simulink model "A5_model_10"  (R2024a)
settings: Solver=VariableStepAuto  StartTime=0.0  StopTime=10  FixedStep=0.00001  MaxStep=1e-3  RelTol=1e-3
values from neighbouring files (symbols this model uses):
  a = data(5)    [A5_41.m]
  A_d = eye(size(A)) + H*(A-(L.*C_Y))    [A5_41.m]
  b = data(6)    [A5_41.m]
  B_d = B * H    [A5_41.m]
  c1 = data(3)    [A5_41.m]
  c2 = data(4)    [A5_41.m]
  h = 0.01    [A5_41.m]
  J_10 = 5220    [A5_41.m]
  K = [S1-temp(2) S2-temp(3) S3-temp(4) S4-temp(5) S5-temp(6)]*Wrtilde*inv(Wr)    [A5_41.m]
  k1 = data(8)    [A5_41.m]
  kr = (-1)/(C_Y*inv(A-B*K)*B)    [A5_41.m]
  L_d = L * H    [A5_41.m]
  m_10 = m+400    [A5_41.m]
  tau = data(7)    [A5_41.m]
  V_10 = 30    [A5_41.m]
settings Model: Creator=jofr  LastModifiedBy=munav
settings SolverCC: AlgebraicLoopSolver=TrustRegion
settings DataIOCC: LimitDataPoints=on  SaveFormat=Array  SignalLoggingSaveFormat=ModelDataLogs  ReturnWorkspaceOutputs=off
settings OptimizationCC: BlockReduction=off  BooleanDataType=off  LifeSpan=inf
settings DebuggingCC: SaveWithParameterizedLinksMsg=none  UnderspecifiedInitializationDetection=Classic  MergeDetectMultiDrivingBlocksExec=none  SignalResolutionControl=TryResolveAllWithWarning  MultiTaskDSMMsg=warning  MultiTaskCondExecSysMsg=none  UnconnectedInputMsg=warning  UnconnectedOutputMsg=warning  UnconnectedLineMsg=warning  SFUnexpectedBacktrackingDiag=warning  SFNoUnconditionalDefaultTransitionDiag=warning  SFExecutionAtInitializationDiag=none  ArithmeticOperatorsInVariantConditions=warning
settings HardwareCC: ProdBitPerPointer=32  ProdBitPerSizeT=32  ProdBitPerPtrDiffT=32  ProdLargestAtomicFloat=None  ProdIntDivRoundTo=Undefined  ProdEndianess=Unspecified  ProdWordSize=32  ProdHWDeviceType=32-bit Generic  TargetUnknown=on
settings ModelReferenceCC: EnableRefExpFcnMdlSchedulingChecks=on  PropagateSignalLabelsOutOfModel=off
settings SFSimCC: SimUseLocalCustomCode=off  CustomCodeUndefinedFunction=UseInterfaceOnly
settings RTWCC: RTWUseLocalCustomCode=off  GPUComputeCapability=3.5  DLArmComputeVersion=19.05
settings CodeAppCC: StateflowObjectComments=on
settings GRTTargetCC: TargetLangStandard=C89/C90 (ANSI)
settings ConfigComp: CovMetricSettings=dw  CovSaveCumulativeToWorkspaceVar=on  CovSaveSingleToWorkspaceVar=on  CovExternalEMLEnable=off

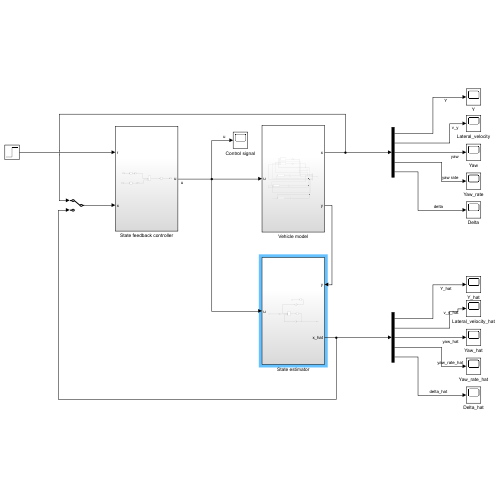
[thumbnail: Simulink's stored preview of the top-level diagram]
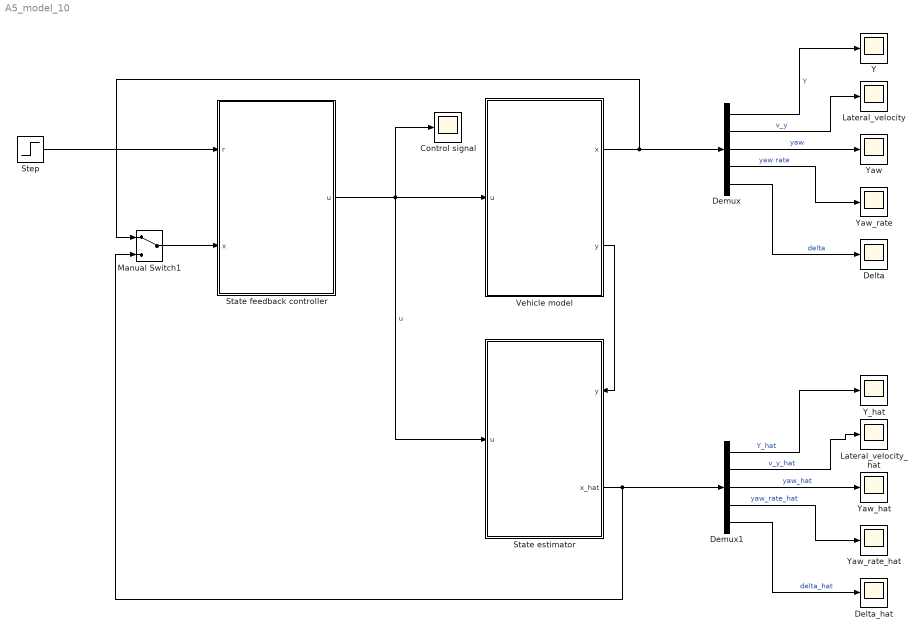
== system A5_model_10 ==
  Control signal : Scope
  Delta : Scope
  Delta_hat : Scope
  Demux : Demux  Outputs=5
  Demux1 : Demux  Outputs=5
  Lateral_velocity : Scope
  Lateral_velocity_hat : Scope
  Manual Switch1 : ManualSwitch
  State estimator : Subsystem
      settings: PortSchema="{\"entries\":[{\"content\":{\"sides\":[{\"content\":{\"connectorIds\":[\"In1\"]},\"type\":\"ConnectorPlacement.EquallySpacedRectSide\",\"uuid\":\"c417f3d4-912d-40bf-9a3a-53ea69fe223c\"},{\"content\":{\"connectorIds\":[\"In2\",\"Out1\"],\"side\":\"RIGHT\"},\"type\":\"ConnectorPlacement.EquallySpacedRectSide\",\"uuid\":\"4e25e672-d4ae-48e6-baf9-37985f0fdcbd\"},{\"content\":{\"connectorIds\":[],\"side\":\"TOP\"},\"type\":\"ConnectorPlacement.EquallySpacedRectSide\",\"uuid\":\"19dfc206-a33d-4b15-9300-bad270a3e9d6\"},{\"content\":{\"connectorIds\":[],\"side\":\"HIDDEN\"},\"type\":\"ConnectorPlacement.EquallySpacedRectSide\",\"uuid\":\"ab455fac-7bff-4c9f-9be5-2f044e5e011f\"}]},\"type\":\"ConnectorPlacement.EquallySpacedConnector\",\"uuid\":\"aea33454-8eab-4b9c-b4de-a2355e2c58aa\"}],\"packageUris\":[\"http://schema.mathworks.com/mf0/Connector/R2020b\"],\"version\":\"1.0\"}"
  State feedback controller : Subsystem
  Step : Step  Time=5  After=3.5  SampleTime=0
  Vehicle model : Subsystem
  Y : Scope
  Y_hat : Scope
  Yaw : Scope
  Yaw_hat : Scope
  Yaw_rate : Scope
  Yaw_rate_hat : Scope
  wires:
  Demux/5 -> Delta/1  "delta"
  Demux/3 -> Yaw/1  "yaw"
  Demux/4 -> Yaw_rate/1  "yaw rate"
  Demux/1 -> Y/1  "Y"
  Demux/2 -> Lateral_velocity/1  "v_y"
  Vehicle model/1(x) -> Manual Switch1/1, Demux/1
  Step/1 -> State feedback controller/1(r)
  Demux1/2 -> Lateral_velocity_hat/1  "v_y_hat"
  Demux1/3 -> Yaw_hat/1  "yaw_hat"
  Demux1/4 -> Yaw_rate_hat/1  "yaw_rate_hat"
  State feedback controller/1(u) -> Control signal/1, State estimator/1(u), Vehicle model/1(u)  "u"
  Demux1/5 -> Delta_hat/1  "delta_hat"
  Demux1/1 -> Y_hat/1  "Y_hat"
  Vehicle model/2(y) -> State estimator/2(y)
  Manual Switch1/1 -> State feedback controller/2(x)
  State estimator/1(x_hat) -> Manual Switch1/2, Demux1/1

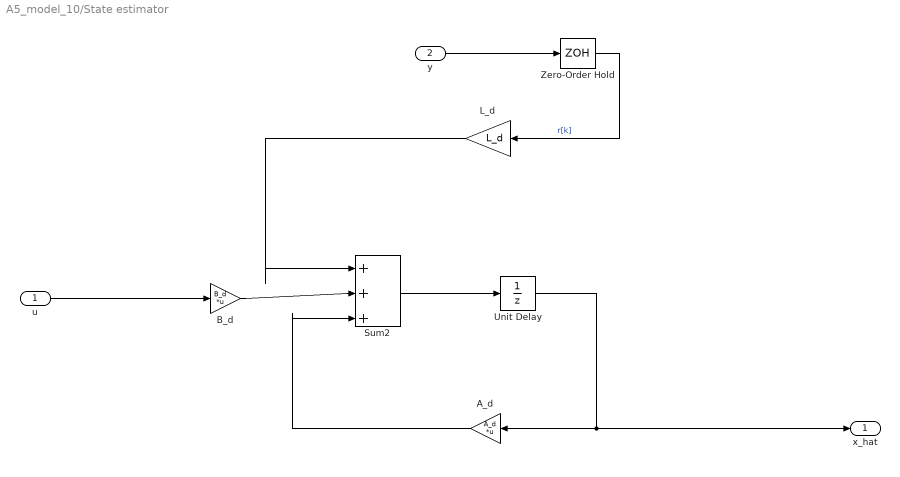
== system A5_model_10/State estimator ==
  u : Inport
  y : Inport  Port=2
  A_d : Gain  Gain=A_d  Multiplication=Matrix(K*u)
  B_d : Gain  Gain=B_d  Multiplication=Matrix(K*u)
  L_d : Gain  Gain=L_d
  Sum2 : Sum  Inputs=|+++
  Unit Delay : UnitDelay  SampleTime=-1  HasFrameUpgradeWarning=on
  Zero-Order Hold : ZeroOrderHold  SampleTime=h
  x_hat : Outport
  wires:
  y/1 -> Zero-Order Hold/1
  u/1 -> B_d/1
  Unit Delay/1 -> x_hat/1, A_d/1
  B_d/1 -> Sum2/2
  L_d/1 -> Sum2/1
  A_d/1 -> Sum2/3
  Sum2/1 -> Unit Delay/1
  Zero-Order Hold/1 -> L_d/1  "r[k]"

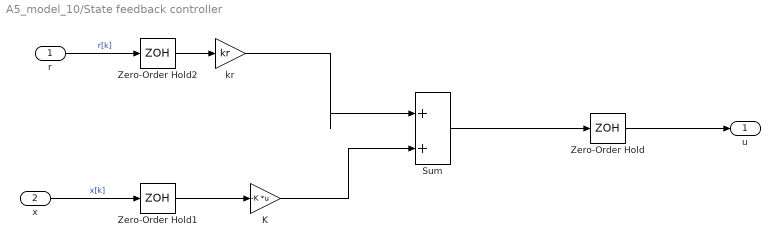
== system A5_model_10/State feedback controller ==
  r : Inport
  x : Inport  Port=2
  K : Gain  Gain=-K  Multiplication=Matrix(K*u)
  Sum : Sum  Inputs=|++
  Zero-Order Hold : ZeroOrderHold  SampleTime=h
  Zero-Order Hold1 : ZeroOrderHold  SampleTime=h
  Zero-Order Hold2 : ZeroOrderHold  SampleTime=h
  kr : Gain  Gain=kr
  u : Outport
  wires:
  x/1 -> Zero-Order Hold1/1  "x[k]"
  r/1 -> Zero-Order Hold2/1  "r[k]"
  Zero-Order Hold/1 -> u/1
  Sum/1 -> Zero-Order Hold/1
  Zero-Order Hold1/1 -> K/1
  Zero-Order Hold2/1 -> kr/1
  kr/1 -> Sum/1
  K/1 -> Sum/2

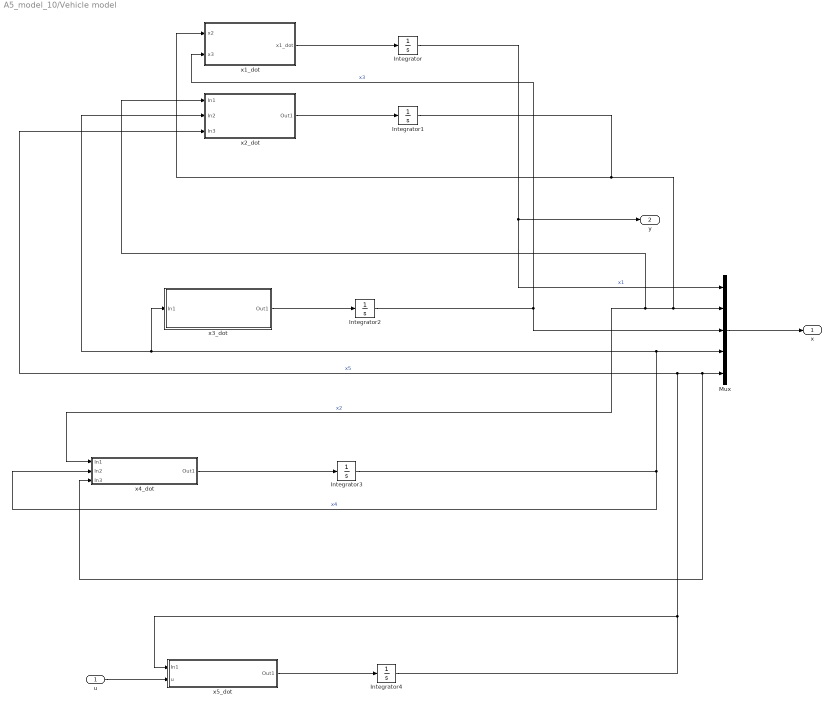
== system A5_model_10/Vehicle model ==
  u : Inport
  Integrator{,1..4} (5 alike) : Integrator
  Mux : Mux  Inputs=5
  x1_dot : Subsystem
  x2_dot : Subsystem
  x3_dot : Subsystem
  x4_dot : Subsystem
  x5_dot : Subsystem
  x : Outport
  y : Outport  Port=2
  wires:
  Integrator3/1 -> Mux/4, x2_dot/2(In2), x3_dot/1(In1), x4_dot/2(In2)  "x4"
  Integrator2/1 -> Mux/3, x1_dot/2(x3)  "x3"
  Integrator/1 -> y/1, Mux/1  "x1"
  Mux/1 -> x/1
  Integrator1/1 -> x4_dot/1(In1), x2_dot/1(In1), Mux/2, x1_dot/1(x2)  "x2"
  Integrator4/1 -> x5_dot/1(In1), x4_dot/3(In3), Mux/5, x2_dot/3(In3)  "x5"
  x1_dot/1(x1_dot) -> Integrator/1
  x2_dot/1(Out1) -> Integrator1/1
  x3_dot/1(Out1) -> Integrator2/1
  x4_dot/1(Out1) -> Integrator3/1
  x5_dot/1(Out1) -> Integrator4/1
  u/1 -> x5_dot/2(u)

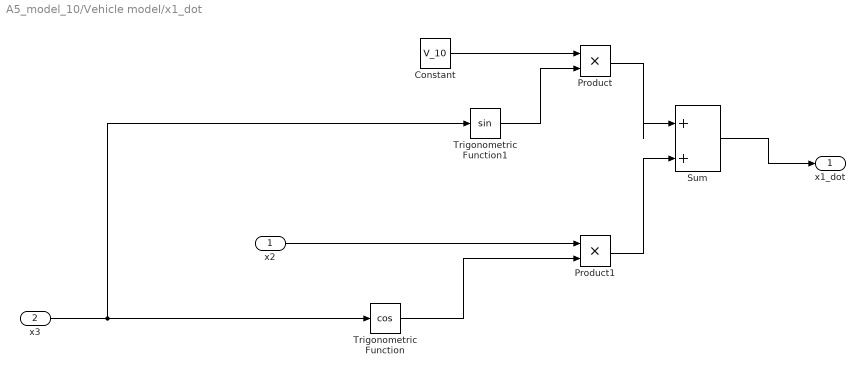
== system A5_model_10/Vehicle model/x1_dot ==
  x2 : Inport
  x3 : Inport  Port=2
  Constant : Constant  Value=V_10
  Product : Product
  Product1 : Product
  Sum : Sum  Inputs=|++
  Trigonometric Function : Trigonometry  Operator=cos
  Trigonometric Function1 : Trigonometry
  x1_dot : Outport
  wires:
  Constant/1 -> Product/1
  Trigonometric Function/1 -> Product1/2
  Sum/1 -> x1_dot/1
  x3/1 -> Trigonometric Function1/1, Trigonometric Function/1
  Product/1 -> Sum/1
  x2/1 -> Product1/1
  Trigonometric Function1/1 -> Product/2
  Product1/1 -> Sum/2

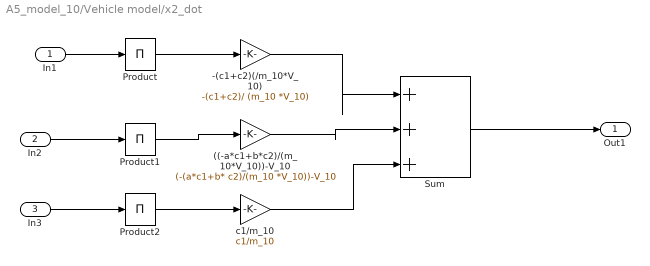
== system A5_model_10/Vehicle model/x2_dot ==
  In1 : Inport
  In2 : Inport  Port=2
  In3 : Inport  Port=3
  ((-a*c1+b*c2)/(m_10*V_10))-V_10 : Gain  Gain=(-(a*c1+b* c2)/(m_10 *V_10))-V_10
  -(c1+c2)(/m_10*V_10) : Gain  Gain=-(c1+c2)/ (m_10 *V_10)
  Product : Product  Inputs=1
  Product1 : Product  Inputs=1
  Product2 : Product  Inputs=1
  Sum : Sum  Inputs=|+++
  c1/m_10 : Gain  Gain=c1/m_10
  Out1 : Outport
  wires:
  -(c1+c2)(/m_10*V_10)/1 -> Sum/1
  ((-a*c1+b*c2)/(m_10*V_10))-V_10/1 -> Sum/2
  c1/m_10/1 -> Sum/3
  Product/1 -> -(c1+c2)(/m_10*V_10)/1
  Product1/1 -> ((-a*c1+b*c2)/(m_10*V_10))-V_10/1
  Product2/1 -> c1/m_10/1
  Sum/1 -> Out1/1
  In1/1 -> Product/1
  In2/1 -> Product1/1
  In3/1 -> Product2/1

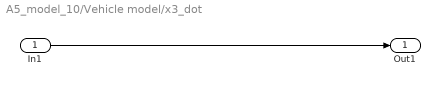
== system A5_model_10/Vehicle model/x3_dot ==
  In1 : Inport
  Out1 : Outport
  wires:
  In1/1 -> Out1/1

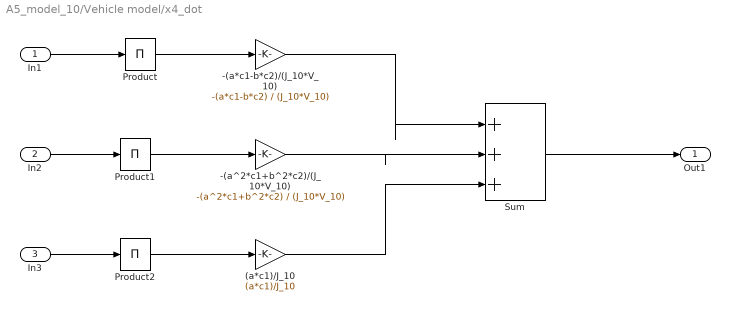
== system A5_model_10/Vehicle model/x4_dot ==
  In1 : Inport
  In2 : Inport  Port=2
  In3 : Inport  Port=3
  (a*c1)/J_10 : Gain  Gain=(a*c1)/J_10
  -(a*c1-b*c2)/(J_10*V_10) : Gain  Gain=-(a*c1-b*c2) / (J_10*V_10)
  -(a^2*c1+b^2*c2)/(J_10*V_10) : Gain  Gain=-(a^2*c1+b^2*c2) / (J_10*V_10)
  Product : Product  Inputs=1
  Product1 : Product  Inputs=1
  Product2 : Product  Inputs=1
  Sum : Sum  Inputs=|+++
  Out1 : Outport
  wires:
  -(a*c1-b*c2)/(J_10*V_10)/1 -> Sum/1
  -(a^2*c1+b^2*c2)/(J_10*V_10)/1 -> Sum/2
  (a*c1)/J_10/1 -> Sum/3
  Sum/1 -> Out1/1
  Product/1 -> -(a*c1-b*c2)/(J_10*V_10)/1
  Product1/1 -> -(a^2*c1+b^2*c2)/(J_10*V_10)/1
  Product2/1 -> (a*c1)/J_10/1
  In1/1 -> Product/1
  In2/1 -> Product1/1
  In3/1 -> Product2/1

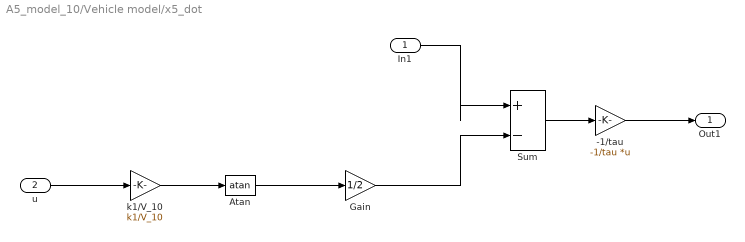
== system A5_model_10/Vehicle model/x5_dot ==
  In1 : Inport
  u : Inport  Port=2
  -1/tau : Gain  Gain=-1/tau  Multiplication=Matrix(K*u)
  Atan : Trigonometry  Operator=atan
  Gain : Gain  Gain=1/2
  Sum : Sum  Inputs=|+-
  k1/V_10 : Gain  Gain=k1/V_10
  Out1 : Outport
  wires:
  k1/V_10/1 -> Atan/1
  u/1 -> k1/V_10/1
  Atan/1 -> Gain/1
  Gain/1 -> Sum/2
  In1/1 -> Sum/1
  Sum/1 -> -1/tau/1
  -1/tau/1 -> Out1/1
